simulink model "Circuit_5"  (R2020b)
settings: Solver=VariableStepAuto  StartTime=0.0  StopTime=10.0  RelTol=1e-3
settings Model: Creator=DELL  LastModifiedBy=DELL

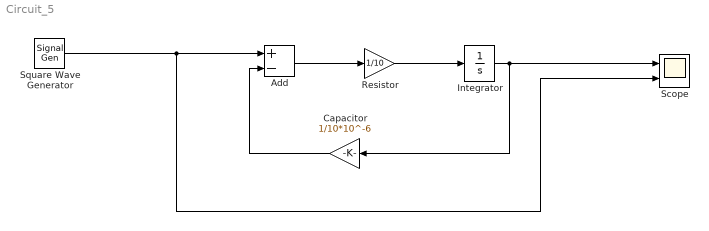
== system Circuit_5 ==
  Add : Sum  Inputs=+-
  Capacitor : Gain  Gain=1/10*10^-6
  Integrator : Integrator  InitialCondition=100*10^-2
  Resistor : Gain  Gain=1/10
  Scope : Scope  NumInputPorts=2
  Square Wave Generator : SignalGenerator  WaveForm=square  Units=rad/sec
  wires:
  Resistor/1 -> Integrator/1
  Integrator/1 -> Capacitor/1, Scope/1
  Add/1 -> Resistor/1
  Square Wave Generator/1 -> Scope/2, Add/1
  Capacitor/1 -> Add/2
